simulink model "vsg"  (R2014a)
settings: Solver=ode45  StartTime=0.0  StopTime=0.5  RelTol=1e-3
undefined symbols (not defined in the file): Ts
libraries: powerlib x13, powerlib_meascontrol x6
settings Model: Creator=ztg  LastModifiedBy=ztg

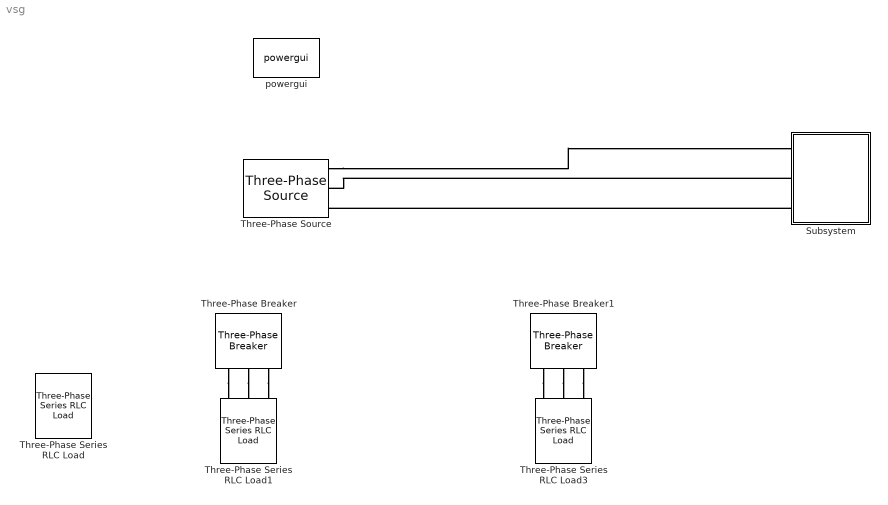
== system vsg ==
  Subsystem : Subsystem  mask{J=0.01, D=20}
      mask TypeOptions J: J/Gain
      mask TypeOptions D: Dp/Gain
  Three-Phase Series RLC Load : powerlib/Elements/Three-Phase Series RLC Load  LConnTagsString=A|B|C  Configuration=Y (grounded)  NominalVoltage=380  NominalFrequency=50  ActivePower=10e3  InductivePower=1  CapacitivePower=1  Measurements=Branch voltages  LoadType=constant Z
  Three-Phase Series RLC Load1 : powerlib/Elements/Three-Phase Series RLC Load  LConnTagsString=A|B|C  Configuration=Y (grounded)  NominalVoltage=380  NominalFrequency=50  ActivePower=1  InductivePower=1  CapacitivePower=5e3  Measurements=Branch voltages  LoadType=constant Z
  Three-Phase Series RLC Load3 : powerlib/Elements/Three-Phase Series RLC Load  LConnTagsString=A|B|C  Configuration=Y (grounded)  NominalVoltage=380  NominalFrequency=50  ActivePower=1  InductivePower=1  CapacitivePower=1  Measurements=Branch voltages  LoadType=constant Z
  Three-Phase Breaker : powerlib/Elements/Three-Phase Breaker  InitialState=open  SwitchA=on  SwitchB=on  SwitchC=on  SwitchTimes=[0.1 0.3]  External=off  BreakerResistance=0.01  SnubberResistance=1e6  SnubberCapacitance=inf  Measurements=None
  Three-Phase Breaker1 : powerlib/Elements/Three-Phase Breaker  InitialState=open  SwitchA=on  SwitchB=on  SwitchC=on  SwitchTimes="[0.5  0.7]"  External=off  BreakerResistance=0.01  SnubberResistance=1e6  SnubberCapacitance=inf  Measurements=None
  Three-Phase Source : powerlib/Electrical Sources/Three-Phase Source  Voltage=380*sqrt(2)  PhaseAngle=0  Frequency=50  InternalConnection=Yg  SpecifyImpedance=off  Resistance=0.8929  Inductance=16.58e-3  ShortCircuitLevel=100e6  BaseVoltage=25e3  XRratio=7  BusType=PV  Pref=10000  Qref=0  Qmin=-inf  Qmax=inf
  powergui : powerlib/powergui  Priority=1  SimulationMode=Discrete  SolverType=Tustin  SampleTime=1e-6  frequency=60  SPID=off  DisableSnubberDevices=off  DisableRonSwitches=off  DisableVfSwitches=off  SwTol=0  Interpol=off  DisplayEquations=off  Ts=0  methode=off  frequencyindice=0  Pbase=100e6  ErrMax=1e-4  Iterations=50  UnitsV=kV  UnitsW=MW  FunctionMessages=off  echomessages=off  HookPort=off  EnableUseOfTLC=off  x0status=blocks  RestoreLinks=warning  ResistiveCurrentMeasurement=off  Frange=[0:2:500]  Ylog=off  Xlog=on  ShowGrid=off  save=off  variable=ZData  structure=ScopeData10  ZoomFFT=off  StartTime=0.1  cycles=1  DisplayStyle=5  fundamental=50  FreqAxis=on  MaxFrequency=1000  frequencyindicesteady=1  RmsSteady=1  display=off
  connections:
  Three-Phase Source/RConn1 -- Subsystem/LConn1
  Subsystem/LConn2 -- Three-Phase Source/RConn2
  Subsystem/LConn3 -- Three-Phase Source/RConn3
  Three-Phase Breaker/RConn3 -- Three-Phase Series RLC Load1/LConn3
  Three-Phase Breaker1/RConn3 -- Three-Phase Series RLC Load3/LConn3
  Three-Phase Breaker1/RConn2 -- Three-Phase Series RLC Load3/LConn2
  Three-Phase Breaker1/RConn1 -- Three-Phase Series RLC Load3/LConn1
  Three-Phase Breaker/RConn2 -- Three-Phase Series RLC Load1/LConn2
  Three-Phase Breaker/RConn1 -- Three-Phase Series RLC Load1/LConn1

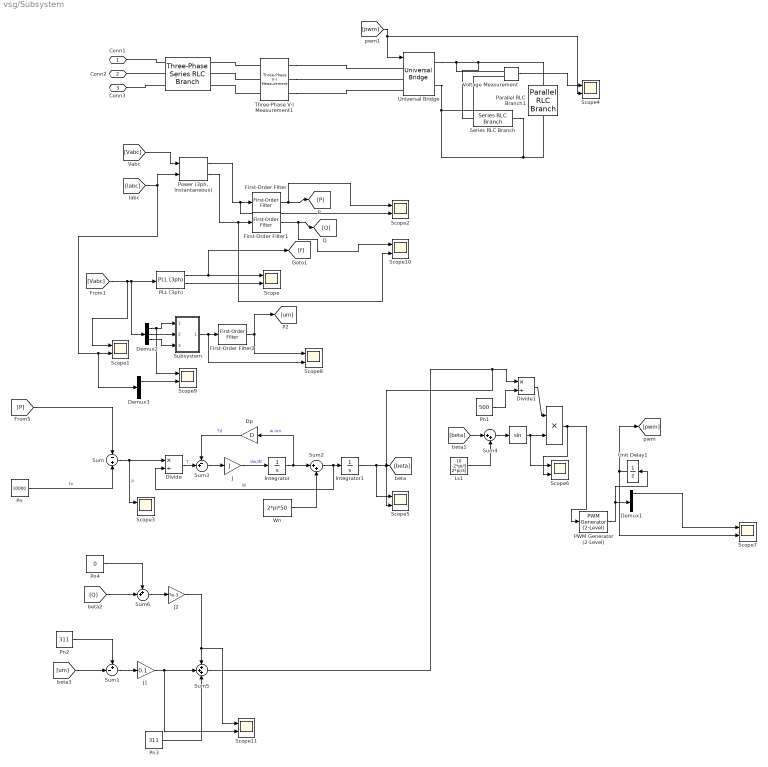
== system vsg/Subsystem ==
  " " : Trigonometry
  "  " : Product
  "                              " : powerlib/Elements/Three-Phase Series RLC Branch  LConnTagsString=A|B|C  RConnTagsString=A|B|C  BranchType=L  Resistance=0.0001  Inductance=5.1e-3  Capacitance=1e-6  Measurements=None
  Demux1 : Demux  Outputs=6
  Demux2 : Demux  Outputs=3
  Demux3 : Demux  Outputs=3
  Divide : Product  Inputs=*/
  Divide1 : Product  Inputs=*/
  Dp : Gain  Gain=D
  First-Order Filter : powerlib_meascontrol/Filters/First-Order Filter  FilterType=Lowpass  Tc=1e-3  Ts=0  Initialize=off  Vac_Init=[0, 0, 50]  Vdc_Init=0  PlotResponse=off  FreqRange="[0,  200,  1]"
  First-Order Filter1 : powerlib_meascontrol/Filters/First-Order Filter  FilterType=Lowpass  Tc=1e-3  Ts=0  Initialize=on  Vac_Init=[0, 0, 50]  Vdc_Init=0  PlotResponse=off  FreqRange="[0,  200,  1]"
  First-Order Filter2 : powerlib_meascontrol/Filters/First-Order Filter  FilterType=Lowpass  Tc=1e-3  Ts=0  Initialize=on  Vac_Init=[0, 0, 50]  Vdc_Init=0  PlotResponse=off  FreqRange="[0,  200,  1]"
  Integrator : Integrator
  Integrator1 : Integrator
  J : Gain  Gain=J
  J1 : Gain  Gain=0.1
  J2 : Gain  Gain=7e-3
  Ls1 : Constant  Value=[0 -2*pi/3 2*pi/3]
  PLL (3ph) : powerlib_meascontrol/PLL/PLL (3ph)  Fmin=45  Par_Init=[0, 50]  ParK=[180, 3200, 1]  TcD=1e-5  MaxRateChangeFreq=12  FilterCutOffFreq=25  Ts=Ts  AGC=on
  PWM Generator (2-Level) : powerlib_meascontrol/Pulse & Signal Generators/PWM Generator (2-Level)  ModulatorType=Three-phase bridge (6 pulses)  ModulatorMode=Unsynchronized  nF=100  Fc=200*50  ModulatingSignals=off  m=0.8  Freq=60  Phase=0  Ts=0
  Parallel RLC Branch1 : powerlib/Elements/Parallel RLC Branch  LConnTagsString=a  RConnTagsString=__new0  BranchType=R  Resistance=100  Inductance=1e-3  SetiL0=off  InitialCurrent=0  Capacitance=1e-6  Setx0=off  InitialVoltage=0  Measurements=None
  Pn : Constant  Value=10000
  Pn1 : Constant  Value=500
  Pn2 : Constant  Value=311
  Pn3 : Constant  Value=311
  Pn4 : Constant  Value=0
  "Power (3ph, Instantaneous)" : powerlib_meascontrol/Measurements/Power (3ph, Instantaneous)
  Scope{,1..11} (12 alike) : Scope  NumInputPorts=2
      Scope settings: YMin=59.9999~0  YMax=60~6.5
      Scope1 settings: YMin=-1200~0  YMax=1200~65
      Scope10 settings: YMin=-1~-3  YMax=1~3  SaveName=ScopeData10
      Scope11 settings: TimeRange=0.5  YMin=-9~-5  YMax=1~35  SaveName=ScopeData11
      Scope2 settings: YMin=6975~6450  YMax=7225~7550  SaveName=ScopeData2
      Scope3 settings: YMin=-9800~-1  YMax=-9000~1  SaveName=ScopeData3
      Scope4 settings: YMin=-50~0  YMax=800~1  SaveName=ScopeData4
      Scope5 settings: YMin=94~-1  YMax=113~1  SaveName=ScopeData5
      Scope6 settings: YMin=-1~-0.8  YMax=1~0.8  SaveName=ScopeData6
      Scope7 settings: TimeRange=0.001051620249093166  YMin=-0.5~-1  YMax=1.5~1  SaveName=ScopeData7
      Scope8 settings: TimeRange=0.8  YMin=0~-1  YMax=500~1  SaveName=ScopeData8
      Scope9 settings: YMin=-350~-22.5  YMax=300~22.5  SaveName=ScopeData9
  Series RLC Branch : powerlib/Elements/Series RLC Branch  LConnTagsString=__new0  RConnTagsString=__new0  BranchType=RLC  Resistance=1  Inductance=1e-9  SetiL0=off  InitialCurrent=0  Capacitance=1e-5  Setx0=off  InitialVoltage=0  Measurements=None
  Subsystem : Subsystem
  Sum : Sum  Inputs=-+
  Sum1 : Sum  Inputs=+-|
  Sum2 : Sum  Inputs=|++
  Sum3 : Sum  Inputs=-+|
  Sum4 : Sum  Inputs=|++
  Sum5 : Sum  Inputs=+++
  Sum6 : Sum  Inputs=++|
  Three-Phase V-I Measurement1 : powerlib/Measurements/Three-Phase V-I Measurement  VoltageMeasurement=phase-to-ground  SetLabelV=on  LabelV=Vabc  Vpu=off  VpuLL=off  CurrentMeasurement=yes  SetLabelI=on  LabelI=Iabc  Ipu=off  Pbase=100e6  Vbase=500e3  OutputType=Complex  PhasorSimulation=off  PSBequivalent=0
  Unit Delay1 : UnitDelay  SampleTime=Ts
  Universal Bridge : powerlib/Power Electronics/Universal Bridge  Arms=3  SnubberResistance=1e5  SnubberCapacitance=inf  Device=IGBT / Diodes  Ron=1e-3  Lon=0  ForwardVoltages="[  0  0  ]"  ForwardVoltage=0  GTOparameters=[ 10e-6 , 20e-6 ]  IGBTparameters=[ 1e-6 , 2e-6 ]  Measurements=None  Measurements_2=None  converterType=Rectifier
  Voltage Measurement : powerlib/Measurements/Voltage Measurement  PhasorSimulation=off  OutputType=Complex  PSBequivalent=0
  Wn : Constant  Value=2*pi*50
  Conn1 : PMIOPort  Port=1  Side=Left
  Conn2 : PMIOPort  Port=2  Side=Left
  Conn3 : PMIOPort  Port=3  Side=Left
  wires:
  [Vabc] -> Demux2/1, PLL (3ph)/1, Scope1/1
  PLL (3ph)/1 -> [f], Scope/1
  PLL (3ph)/2 -> Scope/2
  [Vabc] -> "Power (3ph, Instantaneous)"/1
  [Iabc] -> "Power (3ph, Instantaneous)"/2, Demux3/1, Scope1/2
  "Power (3ph, Instantaneous)"/1 -> Scope2/2, First-Order Filter/1
  "Power (3ph, Instantaneous)"/2 -> Scope10/2, First-Order Filter1/1
  Voltage Measurement/1 -> Scope4/1
  [P] -> Sum/1
  Pn/1 -> Sum/2  "fn"
  Sum/1 -> Divide/1, Scope3/1  "P"
  J/1 -> Integrator/1  "dw/dt"
  Wn/1 -> Sum2/2
  Dp/1 -> Sum3/1  "Td"
  Divide/1 -> Sum3/2  "T"
  Sum3/1 -> J/1
  Sum2/1 -> Divide/2, Integrator1/1  "W"
  Integrator1/1 -> Scope5/1, [beta]
  [pwm] -> Scope4/2, Universal Bridge/1
  Sum4/1 -> " "/1
  [beta] -> Sum4/1
  Ls1/1 -> Sum4/2
  " "/1 -> Scope6/1, "  "/2
  Integrator/1 -> Sum2/1, Dp/1  "w-wn"
  "  "/1 -> Scope6/2, PWM Generator (2-Level)/1
  PWM Generator (2-Level)/1 -> Unit Delay1/1, Demux1/1
  Demux1/1 -> Scope7/1
  Demux2/1 -> Scope9/1, Subsystem/1(In2)
  Demux2/2 -> Subsystem/2(In1)
  Demux2/3 -> Subsystem/3(In3)
  Subsystem/1(Out1) -> Scope8/2, First-Order Filter2/1
  Unit Delay1/1 -> [pwm], Scope7/2
  Sum5/1 -> Scope5/2, Divide1/1
  Divide1/1 -> "  "/1
  Pn1/1 -> Divide1/2
  Pn2/1 -> Sum1/1
  [um] -> Sum1/2
  Sum1/1 -> J1/1
  Pn4/1 -> Sum6/1
  [Q] -> Sum6/2
  Sum6/1 -> J2/1
  J1/1 -> Scope11/2, Sum5/2
  J2/1 -> Scope11/1, Sum5/1
  Pn3/1 -> Sum5/3
  First-Order Filter1/1 -> Scope10/1, [Q]
  First-Order Filter/1 -> Scope2/1, [P]
  Demux3/1 -> Scope9/2
  First-Order Filter2/1 -> Scope8/1, [um]
  connections:
  Universal Bridge/RConn1 -- Voltage Measurement/LConn1 -- Series RLC Branch/LConn1 -- Parallel RLC Branch1/LConn1
  Universal Bridge/RConn2 -- Voltage Measurement/LConn2 -- Series RLC Branch/RConn1 -- Parallel RLC Branch1/RConn1
  "                              "/LConn1 -- Conn1/RConn1
  "                              "/LConn2 -- Conn2/RConn1
  "                              "/LConn3 -- Conn3/RConn1
  Three-Phase V-I Measurement1/RConn1 -- Universal Bridge/LConn1
  Three-Phase V-I Measurement1/RConn2 -- Universal Bridge/LConn2
  Three-Phase V-I Measurement1/RConn3 -- Universal Bridge/LConn3
  Three-Phase V-I Measurement1/LConn1 -- "                              "/RConn1
  Three-Phase V-I Measurement1/LConn2 -- "                              "/RConn2
  Three-Phase V-I Measurement1/LConn3 -- "                              "/RConn3

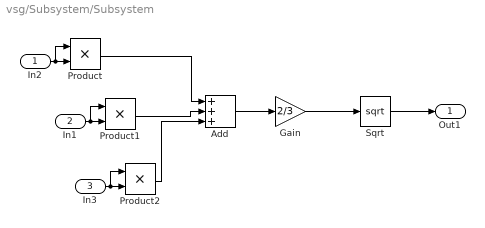
== system vsg/Subsystem/Subsystem ==
  In2 : Inport
  In1 : Inport  Port=2
  In3 : Inport  Port=3
  Add : Sum  Inputs=+++
  Gain : Gain  Gain=2/3
  Product : Product
  Product1 : Product
  Product2 : Product
  Sqrt : Sqrt  SaturateOnIntegerOverflow=on
  Out1 : Outport
  wires:
  In2/1 -> Product/1, Product/2
  In1/1 -> Product1/1, Product1/2
  Product1/1 -> Add/2
  In3/1 -> Product2/1, Product2/2
  Product2/1 -> Add/3
  Product/1 -> Add/1
  Add/1 -> Gain/1
  Sqrt/1 -> Out1/1
  Gain/1 -> Sqrt/1
